simulink model "VVI"  (R2022a)
settings: Solver=FixedStepAuto  StartTime=0.0  StopTime=1  FixedStep=1e-3  RelTol=1e-3  EnableMultiTasking=on
undefined symbols (not defined in the file or in its folder): D1, D10, D11, D12, D13, D2, D3, D4, D5, D7, D8, D9, PTA0, PTA1, PTA2, PTB23, PTB9, PTC17, PTC3, PTC4, PTD0, PTD1, PTD2, PTD3
libraries: frdmk64flib x14
settings Model: ExtModeTrigDuration=5  Creator=anand  LastModifiedBy=anand
settings OptimizationCC: EnhancedBackFolding=on  PassReuseOutputArgsAs=Individual arguments  ZeroExternalMemoryAtStartup=off  ZeroInternalMemoryAtStartup=off  MaxStackSize=64  OptimizeBlockOrder=speed  DifferentSizesBufferReuse=on  OptimizationCustomize=off  EfficientTunableParamExpr=on
settings DebuggingCC: ParameterTunabilityLossMsg=error  SFUnusedDataAndEventsDiag=none
settings HardwareCC: ProdBitPerPointer=32  ProdBitPerSizeT=32  ProdBitPerPtrDiffT=32  ProdLargestAtomicInteger=Long  ProdLargestAtomicFloat=Double  ProdWordSize=32  ProdHWDeviceType=ARM Compatible->ARM Cortex
settings SFSimCC: MATLABDynamicMemAlloc=off
settings RTWCC: SystemTargetFile=ert.tlc  HardwareBoard=NXP FRDM-K64F  TLCOptions="-aInlineSetEventsForThisBaseRateFcn=TLC_FALSE -aSuppressMultiTaskScheduler=TLC_FALSE  -aRateBasedStepFcn=0"  TemplateMakefile=ert_default_tmf  Toolchain=GNU Tools for ARM Embedded Processors
settings CodeAppCC: ForceParamTrailComments=on  IgnoreCustomStorageClasses=off  OperatorAnnotations=on  SimulinkDataObjDesc=on  SFDataObjDesc=on  InsertBlockDesc=on
settings ERTTargetCC: ExtModeTransport=4  ExtModeMexFile=sendToCommService

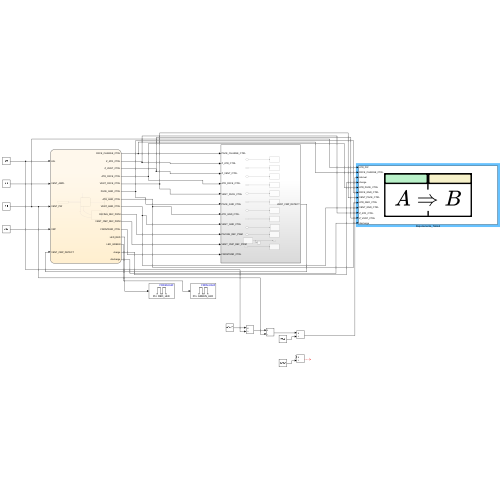
[thumbnail: Simulink's stored preview of the top-level diagram]
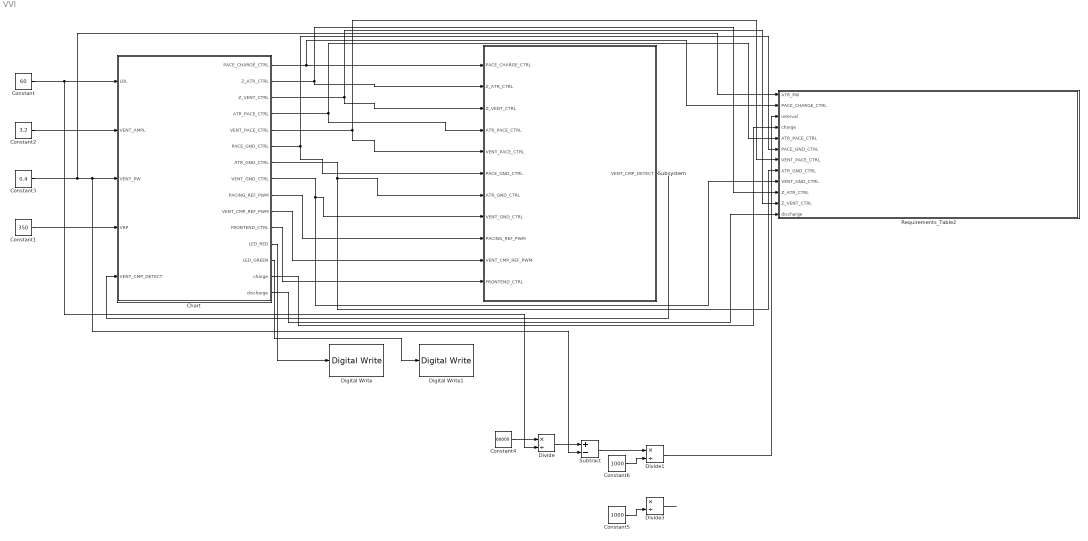
== system VVI ==
  Chart : Stateflow chart  TreatAsAtomicUnit=on
  Constant : Constant  Value=60
  Constant1 : Constant  Value=350
  Constant2 : Constant  Value=3.2
  Constant3 : Constant  Value=0.4
  Constant4 : Constant  Value=60000
  Constant5 : Constant  Value=1000
  Constant6 : Constant  Value=1000
  Digital Write : frdmk64flib/Digital Write  Whichpin=RED_LED
  Digital Write1 : frdmk64flib/Digital Write  Whichpin=GREEN_LED
  Divide : Product  Inputs=*/
  Divide1 : Product  Inputs=*/
  Divide3 : Product  Inputs=*/
  Requirements_Table2 : Requirements Table  TreatAsAtomicUnit=on
  Subsystem : Subsystem
  Subtract : Sum  Inputs=+-
  wires:
  Chart/9(PACING_REF_PWM) -> Subsystem/9(PACING_REF_PWM)
  Constant3/1 -> Requirements_Table2/1(ATR_PW), Subtract/2, Chart/3(VENT_PW)
  Chart/10(VENT_CMP_REF_PWM) -> Subsystem/10(VENT_CMP_REF_PWM)
  Chart/8(VENT_GND_CTRL) -> Requirements_Table2/9(VENT_GND_CTRL), Subsystem/8(VENT_GND_CTRL)
  Constant1/1 -> Chart/4(VRP)
  Chart/4(ATR_PACE_CTRL) -> Subsystem/4(ATR_PACE_CTRL), Requirements_Table2/5(ATR_PACE_CTRL)
  Constant2/1 -> Chart/2(VENT_AMPL)
  Subsystem/1(VENT_CMP_DETECT) -> Chart/5(VENT_CMP_DETECT)
  Chart/5(VENT_PACE_CTRL) -> Subsystem/5(VENT_PACE_CTRL), Requirements_Table2/7(VENT_PACE_CTRL)
  Chart/11(FRONTEND_CTRL) -> Subsystem/11(FRONTEND_CTRL)
  Chart/2(Z_ATR_CTRL) -> Subsystem/2(Z_ATR_CTRL), Requirements_Table2/10(Z_ATR_CTRL)
  Chart/3(Z_VENT_CTRL) -> Subsystem/3(Z_VENT_CTRL), Requirements_Table2/11(Z_VENT_CTRL)
  Chart/6(PACE_GND_CTRL) -> Subsystem/6(PACE_GND_CTRL), Requirements_Table2/6(PACE_GND_CTRL)
  Chart/7(ATR_GND_CTRL) -> Requirements_Table2/8(ATR_GND_CTRL), Subsystem/7(ATR_GND_CTRL)
  Chart/1(PACE_CHARGE_CTRL) -> Requirements_Table2/2(PACE_CHARGE_CTRL), Subsystem/1(PACE_CHARGE_CTRL)
  Constant/1 -> Divide/2, Chart/1(LRL)
  Chart/12(LED_RED) -> Digital Write/1
  Chart/13(LED_GREEN) -> Digital Write1/1
  Divide3/1 -> ?
  Constant4/1 -> Divide/1
  Subtract/1 -> Divide1/1
  Divide/1 -> Subtract/1
  Constant6/1 -> Divide1/2
  Constant5/1 -> Divide3/2
  Divide1/1 -> Requirements_Table2/3(interval)
  Chart/14(charge) -> Requirements_Table2/4(charge)
  Chart/15(discharge) -> Requirements_Table2/12(discharge)

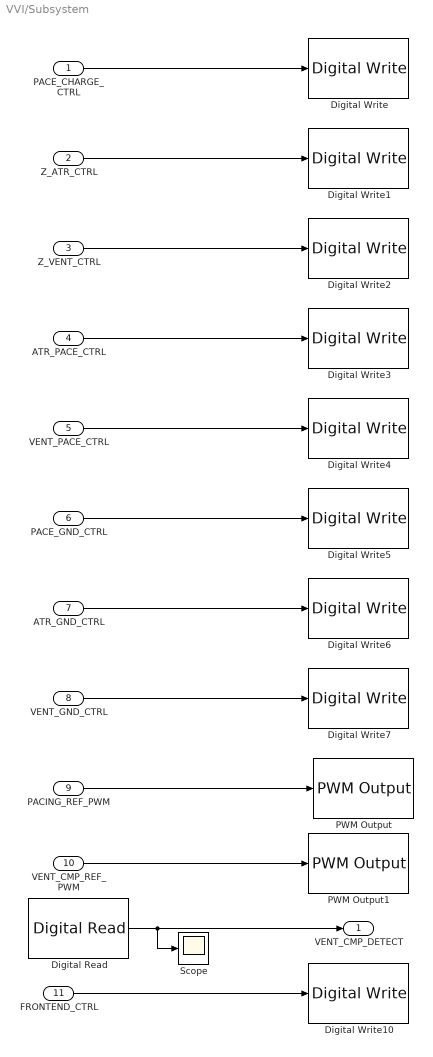
== system VVI/Subsystem ==
  PACE_CHARGE_CTRL : Inport  OutDataTypeStr=boolean
  Z_ATR_CTRL : Inport  Port=2  OutDataTypeStr=boolean
  Z_VENT_CTRL : Inport  Port=3
  ATR_PACE_CTRL : Inport  Port=4
  VENT_PACE_CTRL : Inport  Port=5
  PACE_GND_CTRL : Inport  Port=6
  ATR_GND_CTRL : Inport  Port=7
  VENT_GND_CTRL : Inport  Port=8
  PACING_REF_PWM : Inport  Port=9
  VENT_CMP_REF_PWM : Inport  Port=10
  FRONTEND_CTRL : Inport  Port=11
  Digital Read : frdmk64flib/Digital Read  Whichpin=PTC17 (D1)  SampleTime=-1
  Digital Write : frdmk64flib/Digital Write  Whichpin=PTB9 (D2)
  Digital Write1 : frdmk64flib/Digital Write  Whichpin=PTB23 (D4)
  Digital Write10 : frdmk64flib/Digital Write  Whichpin=PTD1 (D13)
  Digital Write2 : frdmk64flib/Digital Write  Whichpin=PTC3 (D7)
  Digital Write3 : frdmk64flib/Digital Write  Whichpin=PTA0 (D8)
  Digital Write4 : frdmk64flib/Digital Write  Whichpin=PTC4 (D9)
  Digital Write5 : frdmk64flib/Digital Write  Whichpin=PTD0 (D10)
  Digital Write6 : frdmk64flib/Digital Write  Whichpin=PTD2 (D11)
  Digital Write7 : frdmk64flib/Digital Write  Whichpin=PTD3 (D12)
  PWM Output : frdmk64flib/PWM Output  Whichpin=PTA2 (D5)  InitialFrequency=2000  InitialDutyCycle=0
  PWM Output1 : frdmk64flib/PWM Output  Whichpin=PTA1 (D3)  InitialFrequency=2000  InitialDutyCycle=0
  Scope : Scope
  VENT_CMP_DETECT : Outport  OutDataTypeStr=boolean
  wires:
  PACE_CHARGE_CTRL/1 -> Digital Write/1
  Z_ATR_CTRL/1 -> Digital Write1/1
  Z_VENT_CTRL/1 -> Digital Write2/1
  ATR_PACE_CTRL/1 -> Digital Write3/1
  VENT_PACE_CTRL/1 -> Digital Write4/1
  PACE_GND_CTRL/1 -> Digital Write5/1
  ATR_GND_CTRL/1 -> Digital Write6/1
  VENT_GND_CTRL/1 -> Digital Write7/1
  PACING_REF_PWM/1 -> PWM Output/1
  VENT_CMP_REF_PWM/1 -> PWM Output1/1
  Digital Read/1 -> Scope/1, VENT_CMP_DETECT/1
  FRONTEND_CTRL/1 -> Digital Write10/1

== stateflow chart VVI/Chart ==
  state CHARGING
    entry:
    %CHARGING C22
    charge = true;
    discharge = false;
    FRONTEND_CTRL = true;
    ATR_PACE_CTRL = false;
    VENT_PACE_CTRL = false;
    PACING_REF_PWM = 90;
    PACE_CHARGE_CTRL = true;
    VENT_CMP_REF_PWM = 75;
    LED_RED = false;
    LED_GREEN = false;
  state PACE_ATR
    entry:
    charge = false;
    discharge = false;
    PACE_CHARGE_CTRL = false;
    PACE_GND_CTRL = true;
    ATR_PACE_CTRL = false;
    ATR_GND_CTRL = false;
    Z_ATR_CTRL = false;
    Z_VENT_CTRL = false;
    VENT_GND_CTRL = false;
    VENT_PACE_CTRL = true;
    LED_GREEN = true;
  state Ventricular_Refractory_Period_Post_Sensing
    entry:
    LED_RED = true;
  state DISCHARGING
    entry:
    %DISCHARGING C21
    charge = false;
    discharge = true;
    PACE_GND_CTRL = true;
    VENT_PACE_CTRL = false;
    Z_ATR_CTRL = false;
    Z_VENT_CTRL = false;
    ATR_PACE_CTRL = false;
    ATR_GND_CTRL = false;
    VENT_GND_CTRL = true;
  (default) -> CHARGING : {delta = 0; sensing = 0}
  CHARGING -> Ventricular_Refractory_Period_Post_Sensing [order 1] : [VENT_CMP_DETECT == true]
  CHARGING -> PACE_ATR [order 2] : [after(60000/LRL-delta-VENT_PW, msec)]
  Ventricular_Refractory_Period_Post_Sensing -> CHARGING : [after(VRP+35,msec)]{delta = VRP; sensing = 1}
  (junction 103) -> CHARGING : [after(1, msec)]{delta = 0; sensing = 0}
  (junction 101) -> CHARGING : [after(VRP,msec)]{delta = VRP}
  PACE_ATR -> DISCHARGING : [after(VENT_PW,msec)]
  DISCHARGING -> (junction 101) [order 1] : [sensing == 0]
  DISCHARGING -> (junction 103) [order 2] : [sensing == 1]
  data: LRL input; VENT_AMPL input; VENT_PW input; PACE_CHARGE_CTRL output boolean =true; Z_ATR_CTRL output =false; Z_VENT_CTRL output =false; ATR_PACE_CTRL output =false; VENT_PACE_CTRL output =true; PACE_GND_CTRL output =true; ATR_GND_CTRL output =true; VENT_GND_CTRL output =false; PACING_REF_PWM output; VRP input; VENT_CMP_DETECT input boolean size=[1,1]; VENT_CMP_REF_PWM output; delta local double; FRONTEND_CTRL output; sensing local; LED_RED output; LED_GREEN output; charge output; discharge output

== stateflow chart VVI/Requirements_Table2 ==
  (default) -> (junction 1073742982)
  (junction 1073742982) -> (junction 1073742983) : {
      | % SF_REQ_REV_07
      | }
  (junction 1073742983) -> (junction 1073742985) : {
      | % HEADER_ASSIGNMENTS
      |
      | }
  (junction 1073742985) -> (junction 1073742987) : {
      | % START_A_4
      | }
  (junction 1073742987) -> (junction 1073742989) : {
      | }
  (junction 1073742989) -> (junction 1073742991)
  (junction 1073742991) -> (junction 1073742993) : {
      | }
  (junction 1073742993) -> (junction 1073742995) : {
      | % END_A_4
      | }
  (junction 1073742995) -> (junction 1073742997) : {
      | % START_R_16
      | }
  (junction 1073742997) -> (junction 1073742999) : {
      | }
  (junction 1073742999) -> (junction 1073743001)
  (junction 1073743001) -> (junction 1073743003) [order 1] : [(charge == true && discharge == false && t<(interval))]
  (junction 1073743001) -> (junction 1073743009) [order 2]
  (junction 1073743003) -> (junction 1073743005) : {
      | reqtable_postcondition((PACE_GND_CTRL == true && VENT_PACE_CTRL == false && Z_ATR_CTRL == false && Z_VENT_CTRL == false && ATR_PACE_CTRL == false && ATR_GND_CTRL == true && VENT_GND_CTRL == false && PACE_CHARGE_CTRL == true ), 'R:1');
      |
      |
      | }
  (junction 1073743005) -> (junction 1073743007) : {
      | }
  (junction 1073743007) -> (junction 1073743009)
  (junction 1073743009) -> (junction 1073743011)
  (junction 1073743011) -> (junction 1073743013) : {
      | % END_R_16
      | }
  (junction 1073743013) -> (junction 1073743015) : {
      | % START_R_19
      | }
  (junction 1073743015) -> (junction 1073743017) : {
      | }
  (junction 1073743017) -> (junction 1073743019)
  (junction 1073743019) -> (junction 1073743021) [order 1] : [( charge == false && (interval)<=t<= (interval+ATR_PW))]
  (junction 1073743019) -> (junction 1073743027) [order 2]
  (junction 1073743021) -> (junction 1073743023) : {
      | reqtable_postcondition((PACE_CHARGE_CTRL == false && PACE_GND_CTRL == true && PACE_GND_CTRL == true && VENT_PACE_CTRL == true && Z_ATR_CTRL == false && Z_VENT_CTRL == false && ATR_PACE_CTRL == false && ATR_GND_CTRL == false && VENT_GND_CTRL == false), 'R:2');
      |
      |
      | }
  (junction 1073743023) -> (junction 1073743025) : {
      | }
  (junction 1073743025) -> (junction 1073743027)
  (junction 1073743027) -> (junction 1073743029)
  (junction 1073743029) -> (junction 1073743031) : {
      | % END_R_19
      | }
  (junction 1073743031) -> (junction 1073743033) : {
      | % START_R_13
      | }
  (junction 1073743033) -> (junction 1073743035) : {
      | }
  (junction 1073743035) -> (junction 1073743037)
  (junction 1073743037) -> (junction 1073743039) [order 1] : [( charge == true && t > interval)]
  (junction 1073743037) -> (junction 1073743045) [order 2]
  (junction 1073743039) -> (junction 1073743041) : {
      | reqtable_postcondition((PACE_GND_CTRL == true && VENT_PACE_CTRL == false && Z_ATR_CTRL == false && Z_VENT_CTRL == false && ATR_PACE_CTRL == false && ATR_GND_CTRL == true && VENT_GND_CTRL == false && PACE_CHARGE_CTRL == true ), 'R:3');
      |
      |
      | }
  (junction 1073743041) -> (junction 1073743043) : {
      | }
  (junction 1073743043) -> (junction 1073743045)
  (junction 1073743045) -> (junction 1073743047)
  (junction 1073743047) -> (junction 1073743049) : {
      | % END_R_13
      | }
  data: ATR_PW input double; PACE_CHARGE_CTRL input; interval input; charge input boolean; ATR_PACE_CTRL input boolean; PACE_GND_CTRL input boolean; VENT_PACE_CTRL input boolean; ATR_GND_CTRL input boolean; VENT_GND_CTRL input boolean; Z_ATR_CTRL input boolean; Z_VENT_CTRL input boolean; discharge input boolean
